simulink model "Observer_design_acceleration_tau"  (R2016b)
settings: Solver=FixedStepAuto  StartTime=0.0  StopTime=5  FixedStep=0.00001  RelTol=1e-3
settings Model: Creator=emilio  LastModifiedBy=danielesmn

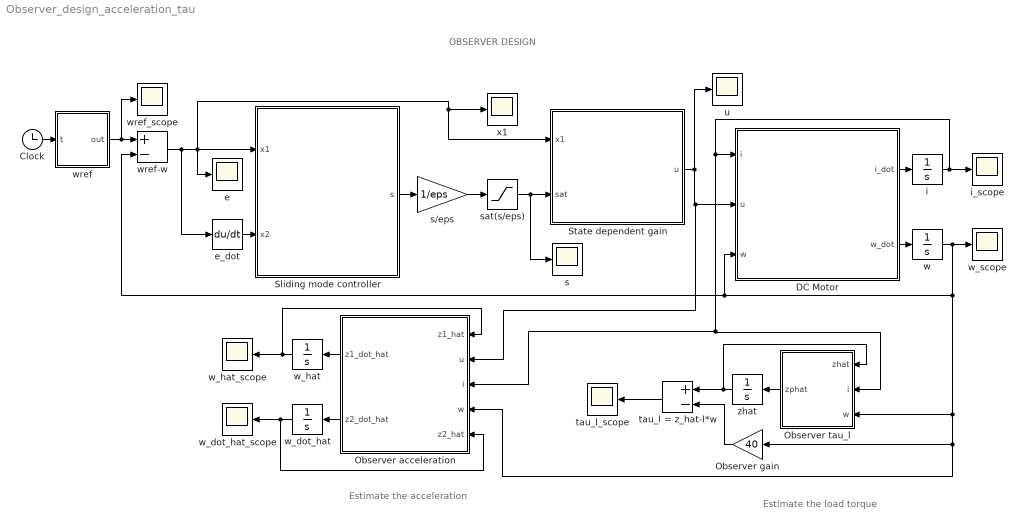
== system Observer_design_acceleration_tau ==
  note: Estimate the acceleration
  note: Estimate the load torque
  note: OBSERVER DESIGN
  Clock : Clock
  DC Motor : MATLAB Function  TreatAsAtomicUnit=on
  Observer acceleration : MATLAB Function  TreatAsAtomicUnit=on
  Observer gain : Gain  Gain=40
  Observer tau_l : MATLAB Function  TreatAsAtomicUnit=on
  Sliding mode controller : MATLAB Function  TreatAsAtomicUnit=on
  State dependent gain : MATLAB Function  TreatAsAtomicUnit=on
  e : Scope
  e_dot : Derivative
  i : Integrator
  i_scope : Scope
  s : Scope
  s/eps : Gain  Gain=1/eps
  sat(s/eps) : Saturate  UpperLimit=1  LowerLimit=-1  ZeroCross=off
  tau_l = z_hat-l*w : Sum  Inputs=+-
  tau_l_scope : Scope
  u : Scope
  w : Integrator
  w_dot_hat : Integrator  InitialCondition=1
  w_dot_hat_scope : Scope
  w_hat : Integrator  InitialCondition=1
  w_hat_scope : Scope
  w_scope : Scope
  wref : MATLAB Function  TreatAsAtomicUnit=on
  wref-w : Sum  Inputs=+-
  wref_scope : Scope
  x1 : Scope
  zhat : Integrator  InitialCondition=0.01
  wires:
  wref-w/1 -> e_dot/1, x1/1, State dependent gain/1(x1), e/1, Sliding mode controller/1(x1)
  wref/1(out) -> wref_scope/1, wref-w/1
  e_dot/1 -> Sliding mode controller/2(x2)
  Clock/1 -> wref/1(t)
  DC Motor/2(w_dot) -> w/1
  w/1 -> Observer tau_l/3(w), Observer acceleration/4(w), Observer gain/1, wref-w/2, DC Motor/3(w), w_scope/1
  i/1 -> i_scope/1, DC Motor/1(i), Observer acceleration/3(i), Observer tau_l/2(i)
  s/eps/1 -> sat(s/eps)/1
  Sliding mode controller/1(s) -> s/eps/1
  State dependent gain/1(u) -> u/1, Observer acceleration/2(u), DC Motor/2(u)
  sat(s/eps)/1 -> s/1, State dependent gain/2(sat)
  Observer tau_l/1(zphat) -> zhat/1
  zhat/1 -> tau_l = z_hat-l*w/1, Observer tau_l/1(zhat)
  Observer gain/1 -> tau_l = z_hat-l*w/2
  DC Motor/1(i_dot) -> i/1
  tau_l = z_hat-l*w/1 -> tau_l_scope/1
  Observer acceleration/1(z1_dot_hat) -> w_hat/1
  Observer acceleration/2(z2_dot_hat) -> w_dot_hat/1
  w_hat/1 -> w_hat_scope/1, Observer acceleration/1(z1_hat)
  w_dot_hat/1 -> Observer acceleration/5(z2_hat), w_dot_hat_scope/1

== matlab function Observer_design_acceleration_tau/State dependent gain ==
  data: x1 input; u output; sat input
function u = SDG(x1, sat)

u0 = 1;
delta = 10;

u = (u0 + delta*abs(x1))*sat;

== matlab function Observer_design_acceleration_tau/Sliding mode controller ==
  data: x1 input; x2 input; s output
function s = SMC(x1, x2)

c = 30;

s = c*x1 + x2;

== matlab function Observer_design_acceleration_tau/Observer tau_l ==
  data: zhat input; i input; zphat output; w input
function zphat = ObsTau_l(zhat, i, w)

kt = 0.008;       %Torque constant (Nm/A)
J = 0.001;        %Inertia of the motor rotor (Kg*m^2)
l = 40;           %Observer gain

zphat = 1/J*(-l*zhat + l^2*w + l*kt*i);

== matlab function Observer_design_acceleration_tau/wref ==
  data: t input; out output
function out = input(t)

if t > 2 && t < 3.5
    out = 1;
else
    out = -1;
end

== matlab function Observer_design_acceleration_tau/DC Motor ==
  data: i_dot output; w_dot output; i input; u input; w input
function [i_dot, w_dot] = Dc_Motor(i, u, w) % i: armature current w: shaft speed

%% Model of the DC Motor

L = 0.001;        %Armature inductance (H)
R = 0.5;          %Armature resistance (Ohm)
kt = 0.008;       %Torque constant (Nm/A)
J = 0.001;        %Inertia of the motor rotor (Kg*m^2)
B = 0.01;         %Coefficient of viscous friction (Nm*s/rad)
lambda0 = 0.001;  %Back electromotive force (EMF) constant (V*s/rad)

tauL = B*w;        %Load torque

i_dot = u/L - R/L*i - lambda0/L*w;      %Electrical part model
w_dot = (kt*i - tauL)/J;              %Mechanical part model

== matlab function Observer_design_acceleration_tau/Observer acceleration ==
  data: z1_hat input; u input; i input; w input; z2_hat input; z1_dot_hat output; z2_dot_hat output
function [z1_dot_hat, z2_dot_hat] = ObsAcc(z1_hat, u, i, w, z2_hat) 

%z1_hat: w_hat, z2_hat: w_dot_hat

L = 0.001;        %Armature inductance (H)
R = 0.5;          %Armature resistance (Ohm)
kt = 0.008;       %Torque constant (Nm/A)
J = 0.001;        %Inertia of the motor rotor (Kg*m^2)
B = 0.01;         %Coefficient of viscous friction (Nm*s/rad)
lambda0 = 0.001;  %Back electromotive force (EMF) constant (V*s/rad)
l1 = 10;          %Observer gain 1
l2 = 10;          %Observer gain 2

z1_dot_hat = z2_hat  - l1*(z1_hat - w);
z2_dot_hat = kt/(J*L)*(u - R*i - lambda0*z1_hat) - l2*(z1_hat - w);
